simulink model "DCT_2D_BAS2008"  (R2015b)
settings: Solver=VariableStepAuto  StartTime=0.0  StopTime=70*st  RelTol=1e-3
values from neighbouring files (symbols this model uses):
  a = 1    [DCT_2d.m]
  a_mux = 2    [DCT_2d.m]
  st = 10/(10*1e6)    (= 1e-06)    [DCT_2d.m]
libraries: xbsIndex_r4 x169
settings Model: Creator=Namalka  LastModifiedBy=Namalka

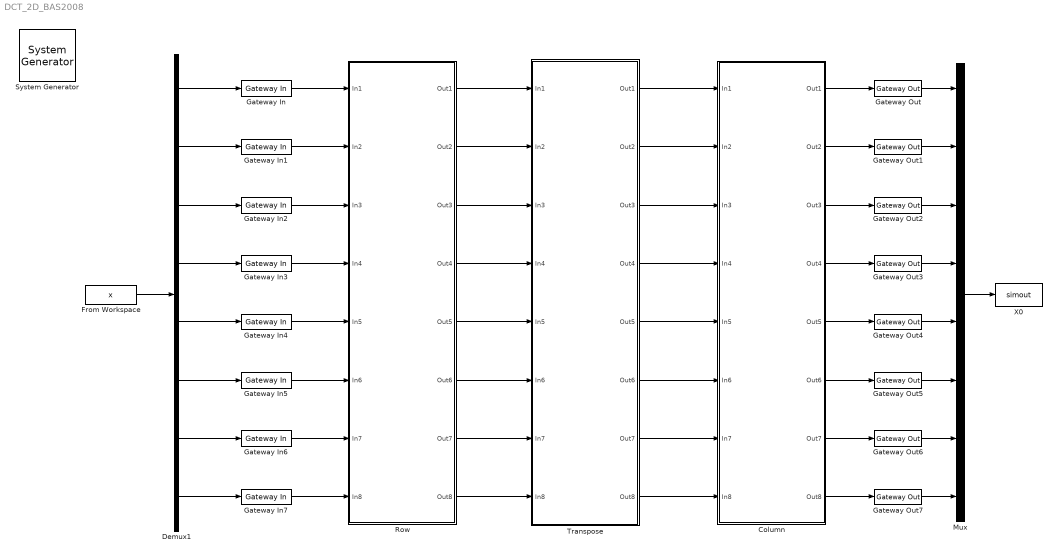
== system DCT_2D_BAS2008 ==
  " System Generator" : xbsIndex_r4/ System Generator  Tag=genX  xilinxfamily=virtex7  part=xc7vx485t  speed=-2  package=ffg1761  synthesis_tool=XST  clock_wrapper=Clock Enables  directory=D:/ISCAS2020/BAS2008/DCT2D  proj_type=Vivado  Synth_file=Vivado Synthesis Defaults  Impl_file=Vivado Implementation Defaults  testbench=off  simulink_period=st  sysclk_period=st*10e6  dcm_input_clock_period=100  incr_netlist=off  trim_vbits=Everywhere in SubSystem  dbl_ovrd=According to Block Masks  core_generation=According to Block Masks  run_coregen=off  deprecated_control=off  eval_field=0  block_type=sysgen
      settings: block_version=10.1
  Column : Subsystem
  Demux1 : Demux  Outputs=8
  From Workspace : FromWorkspace  VariableName=x  SampleTime=0
  Gateway In{,1..7} (8 alike) : xbsIndex_r4/Gateway In  gui_display_data_type=Fixed-point  arith_type="Signed  (2's comp)"  n_bits=W  bin_pt=B  preci_type=Single  exp_width=8  frac_width=24  rows=1  columns=1  quantization="Round  (unbiased: +/- Inf)"  overflow=Saturate  period=st  UseAsADC=off  ADCChannel='1'  interface=None  automatic_assignment=on  address_offset=hex2dec('00')  intf_name=''  intf_description=''  default_value=0  timing_constraint=None  locs_specified=off  LOCs={}  io_standard={}  inherit_from_input=off  hdl_port=on  dbl_ovrd=off  block_type=gatewayin
  Gateway Out{,1..7} (8 alike) : xbsIndex_r4/Gateway Out  inherit_from_input=off  hdl_port=on  rows=1  columns=1  UseAsDAC=off  DACChannel='1'  interface=None  automatic_assignment=on  address_offset=hex2dec('00')  intf_name=''  intf_description=''  timing_constraint=None  locs_specified=off  LOCs={}  io_standard={}  block_type=gatewayout
  Mux : Mux  Inputs=8
  Row : Subsystem
  Transpose : Subsystem
  X0 : ToWorkspace  VariableName=simout  SampleTime=-1
  wires:
  Demux1/1 -> Gateway In/1
  Demux1/2 -> Gateway In1/1
  Demux1/3 -> Gateway In2/1
  Demux1/4 -> Gateway In3/1
  Demux1/5 -> Gateway In4/1
  Demux1/6 -> Gateway In5/1
  Demux1/7 -> Gateway In6/1
  Demux1/8 -> Gateway In7/1
  Gateway In7/1 -> Row/8(In8)
  From Workspace/1 -> Demux1/1
  Gateway In/1 -> Row/1(In1)
  Gateway In6/1 -> Row/7(In7)
  Gateway In1/1 -> Row/2(In2)
  Gateway In2/1 -> Row/3(In3)
  Gateway In3/1 -> Row/4(In4)
  Gateway In4/1 -> Row/5(In5)
  Gateway In5/1 -> Row/6(In6)
  Mux/1 -> X0/1
  Gateway Out7/1 -> Mux/8
  Gateway Out6/1 -> Mux/7
  Gateway Out5/1 -> Mux/6
  Gateway Out4/1 -> Mux/5
  Gateway Out3/1 -> Mux/4
  Gateway Out2/1 -> Mux/3
  Gateway Out1/1 -> Mux/2
  Gateway Out/1 -> Mux/1
  Column/8(Out8) -> Gateway Out7/1
  Column/7(Out7) -> Gateway Out6/1
  Column/1(Out1) -> Gateway Out/1
  Column/2(Out2) -> Gateway Out1/1
  Column/3(Out3) -> Gateway Out2/1
  Column/4(Out4) -> Gateway Out3/1
  Column/6(Out6) -> Gateway Out5/1
  Column/5(Out5) -> Gateway Out4/1
  Transpose/7(Out7) -> Column/7(In7)
  Transpose/1(Out1) -> Column/1(In1)
  Transpose/2(Out2) -> Column/2(In2)
  Transpose/3(Out3) -> Column/3(In3)
  Transpose/4(Out4) -> Column/4(In4)
  Transpose/6(Out6) -> Column/6(In6)
  Transpose/5(Out5) -> Column/5(In5)
  Transpose/8(Out8) -> Column/8(In8)
  Row/7(Out7) -> Transpose/7(In7)
  Row/1(Out1) -> Transpose/1(In1)
  Row/2(Out2) -> Transpose/2(In2)
  Row/3(Out3) -> Transpose/3(In3)
  Row/4(Out4) -> Transpose/4(In4)
  Row/6(Out6) -> Transpose/6(In6)
  Row/5(Out5) -> Transpose/5(In5)
  Row/8(Out8) -> Transpose/8(In8)

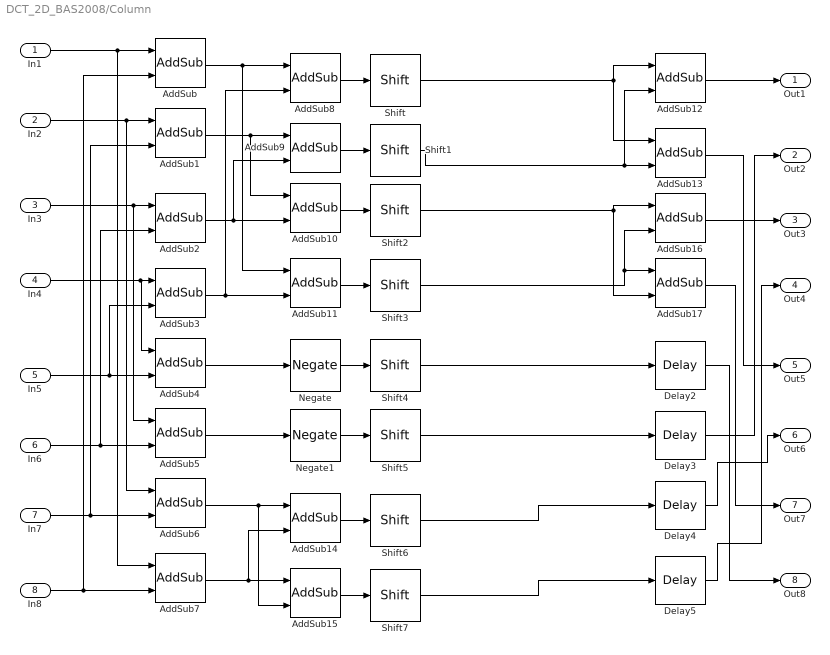
== system DCT_2D_BAS2008/Column ==
  In1 : Inport
  In2 : Inport  Port=2
  In3 : Inport  Port=3
  In4 : Inport  Port=4
  In5 : Inport  Port=5
  In6 : Inport  Port=6
  In7 : Inport  Port=7
  In8 : Inport  Port=8
  AddSub{,1..3,8..9,12,14,16} (9 alike) : xbsIndex_r4/AddSub  mode=Addition  use_carryin=off  use_carryout=off  en=off  latency=a  precision=User Defined  arith_type="Signed  (2's comp)"  n_bits=W  bin_pt=B  quantization="Round  (unbiased: +/- Inf)"  overflow=Saturate  use_behavioral_HDL=off  hw_selection=Fabric  pipelined=off  dbl_ovrd=off  block_type=addsub
  AddSub{4..7,10..11,13,15,17} (9 alike) : xbsIndex_r4/AddSub  mode=Subtraction  use_carryin=off  use_carryout=off  en=off  latency=a  precision=User Defined  arith_type="Signed  (2's comp)"  n_bits=W  bin_pt=B  quantization="Round  (unbiased: +/- Inf)"  overflow=Saturate  use_behavioral_HDL=off  hw_selection=Fabric  pipelined=off  dbl_ovrd=off  block_type=addsub
  Delay{2..5} (4 alike) : xbsIndex_r4/Delay  rst=off  infoeditControl=Selection of Reset will increase slice count due to use of real FFs and instead of SRLs  en=off  latency=a  reg_retiming=off  dbl_ovrd=off  block_type=delay
      settings: infoedit=Hardware notes: A delay line is a chain, each link of which is an SRL16 or SRL32 followed by a flip-flop.
  Negate : xbsIndex_r4/Negate  precision=Full  arith_type=Unsigned  n_bits=16  bin_pt=14  quantization=Truncate  overflow=Wrap  en=off  latency=1  dbl_ovrd=off  block_type=negate
  Negate1 : xbsIndex_r4/Negate  precision=Full  arith_type=Unsigned  n_bits=16  bin_pt=14  quantization=Truncate  overflow=Wrap  en=off  latency=1  dbl_ovrd=off  block_type=negate
  Shift{,1..7} (8 alike) : xbsIndex_r4/Shift  shift_dir=Left  shift_bits=1  en=off  latency=a  precision=Full  arith_type="Signed  (2's comp)"  n_bits=16  bin_pt=14  quantization=Truncate  overflow=Wrap  dbl_ovrd=off  block_type=shift
  Out1 : Outport
  Out2 : Outport  Port=2
  Out3 : Outport  Port=3
  Out4 : Outport  Port=4
  Out5 : Outport  Port=5
  Out6 : Outport  Port=6
  Out7 : Outport  Port=7
  Out8 : Outport  Port=8
  wires:
  In8/1 -> AddSub7/2, AddSub/2
  AddSub8/1 -> Shift/1
  In1/1 -> AddSub/1, AddSub7/1
  In2/1 -> AddSub6/1, AddSub1/1
  In3/1 -> AddSub5/1, AddSub2/1
  In4/1 -> AddSub4/1, AddSub3/1
  In5/1 -> AddSub3/2, AddSub4/2
  In6/1 -> AddSub2/2, AddSub5/2
  In7/1 -> AddSub1/2, AddSub6/2
  AddSub/1 -> AddSub11/1, AddSub8/1
  AddSub1/1 -> AddSub10/1, AddSub9/1
  AddSub2/1 -> AddSub9/2, AddSub10/2
  AddSub3/1 -> AddSub8/2, AddSub11/2
  AddSub9/1 -> Shift1/1
  AddSub11/1 -> Shift3/1
  AddSub4/1 -> Negate/1
  AddSub5/1 -> Negate1/1
  AddSub10/1 -> Shift2/1
  Negate/1 -> Shift4/1
  Negate1/1 -> Shift5/1
  AddSub6/1 -> AddSub15/2, AddSub14/1
  AddSub7/1 -> AddSub15/1, AddSub14/2
  Shift/1 -> AddSub13/1, AddSub12/1
  Shift1/1 -> AddSub12/2, AddSub13/2
  Shift4/1 -> Delay2/1
  Shift5/1 -> Delay3/1
  AddSub14/1 -> Shift6/1
  AddSub15/1 -> Shift7/1
  Shift2/1 -> AddSub17/2, AddSub16/1
  Shift3/1 -> AddSub17/1, AddSub16/2
  AddSub12/1 -> Out1/1
  Shift6/1 -> Delay4/1
  Shift7/1 -> Delay5/1
  AddSub13/1 -> Out5/1
  AddSub16/1 -> Out3/1
  AddSub17/1 -> Out7/1
  Delay2/1 -> Out8/1
  Delay3/1 -> Out2/1
  Delay4/1 -> Out6/1
  Delay5/1 -> Out4/1

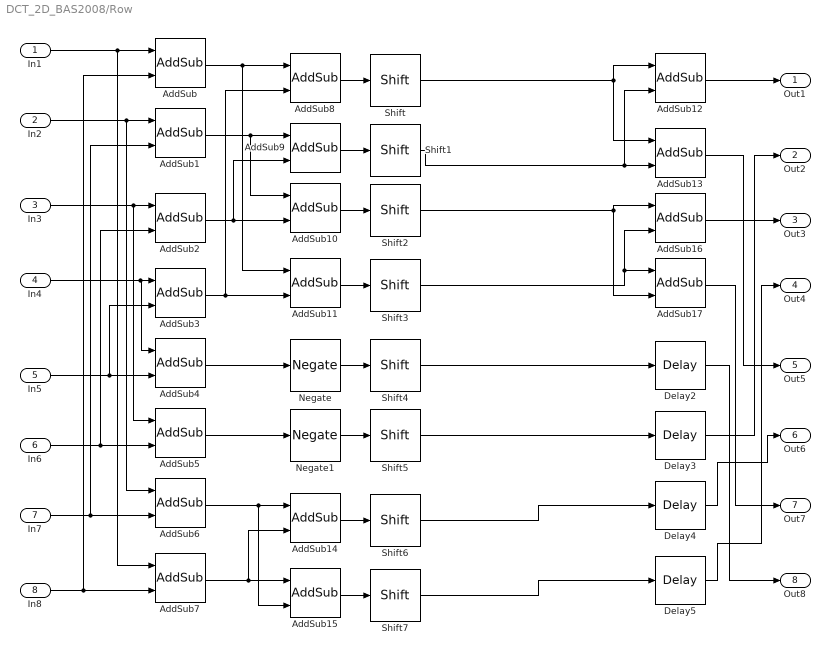
== system DCT_2D_BAS2008/Row ==
  In1 : Inport
  In2 : Inport  Port=2
  In3 : Inport  Port=3
  In4 : Inport  Port=4
  In5 : Inport  Port=5
  In6 : Inport  Port=6
  In7 : Inport  Port=7
  In8 : Inport  Port=8
  AddSub{,1..3,8..9,12,14,16} (9 alike) : xbsIndex_r4/AddSub  mode=Addition  use_carryin=off  use_carryout=off  en=off  latency=a  precision=User Defined  arith_type="Signed  (2's comp)"  n_bits=W  bin_pt=B  quantization="Round  (unbiased: +/- Inf)"  overflow=Saturate  use_behavioral_HDL=off  hw_selection=Fabric  pipelined=off  dbl_ovrd=off  block_type=addsub
  AddSub{4..7,10..11,13,15,17} (9 alike) : xbsIndex_r4/AddSub  mode=Subtraction  use_carryin=off  use_carryout=off  en=off  latency=a  precision=User Defined  arith_type="Signed  (2's comp)"  n_bits=W  bin_pt=B  quantization="Round  (unbiased: +/- Inf)"  overflow=Saturate  use_behavioral_HDL=off  hw_selection=Fabric  pipelined=off  dbl_ovrd=off  block_type=addsub
  Delay{2..5} (4 alike) : xbsIndex_r4/Delay  rst=off  infoeditControl=Selection of Reset will increase slice count due to use of real FFs and instead of SRLs  en=off  latency=a  reg_retiming=off  dbl_ovrd=off  block_type=delay
      settings: infoedit=Hardware notes: A delay line is a chain, each link of which is an SRL16 or SRL32 followed by a flip-flop.
  Negate : xbsIndex_r4/Negate  precision=Full  arith_type=Unsigned  n_bits=16  bin_pt=14  quantization=Truncate  overflow=Wrap  en=off  latency=1  dbl_ovrd=off  block_type=negate
  Negate1 : xbsIndex_r4/Negate  precision=Full  arith_type=Unsigned  n_bits=16  bin_pt=14  quantization=Truncate  overflow=Wrap  en=off  latency=1  dbl_ovrd=off  block_type=negate
  Shift{,1..7} (8 alike) : xbsIndex_r4/Shift  shift_dir=Left  shift_bits=1  en=off  latency=a  precision=Full  arith_type="Signed  (2's comp)"  n_bits=16  bin_pt=14  quantization=Truncate  overflow=Wrap  dbl_ovrd=off  block_type=shift
  Out1 : Outport
  Out2 : Outport  Port=2
  Out3 : Outport  Port=3
  Out4 : Outport  Port=4
  Out5 : Outport  Port=5
  Out6 : Outport  Port=6
  Out7 : Outport  Port=7
  Out8 : Outport  Port=8
  wires:
  In8/1 -> AddSub7/2, AddSub/2
  AddSub8/1 -> Shift/1
  In1/1 -> AddSub/1, AddSub7/1
  In2/1 -> AddSub6/1, AddSub1/1
  In3/1 -> AddSub5/1, AddSub2/1
  In4/1 -> AddSub4/1, AddSub3/1
  In5/1 -> AddSub3/2, AddSub4/2
  In6/1 -> AddSub2/2, AddSub5/2
  In7/1 -> AddSub1/2, AddSub6/2
  AddSub/1 -> AddSub11/1, AddSub8/1
  AddSub1/1 -> AddSub10/1, AddSub9/1
  AddSub2/1 -> AddSub9/2, AddSub10/2
  AddSub3/1 -> AddSub8/2, AddSub11/2
  AddSub9/1 -> Shift1/1
  AddSub11/1 -> Shift3/1
  AddSub4/1 -> Negate/1
  AddSub5/1 -> Negate1/1
  AddSub10/1 -> Shift2/1
  Negate/1 -> Shift4/1
  Negate1/1 -> Shift5/1
  AddSub6/1 -> AddSub15/2, AddSub14/1
  AddSub7/1 -> AddSub15/1, AddSub14/2
  Shift/1 -> AddSub13/1, AddSub12/1
  Shift1/1 -> AddSub12/2, AddSub13/2
  Shift4/1 -> Delay2/1
  Shift5/1 -> Delay3/1
  AddSub14/1 -> Shift6/1
  AddSub15/1 -> Shift7/1
  Shift2/1 -> AddSub17/2, AddSub16/1
  Shift3/1 -> AddSub17/1, AddSub16/2
  AddSub12/1 -> Out1/1
  Shift6/1 -> Delay4/1
  Shift7/1 -> Delay5/1
  AddSub13/1 -> Out5/1
  AddSub16/1 -> Out3/1
  AddSub17/1 -> Out7/1
  Delay2/1 -> Out8/1
  Delay3/1 -> Out2/1
  Delay4/1 -> Out6/1
  Delay5/1 -> Out4/1

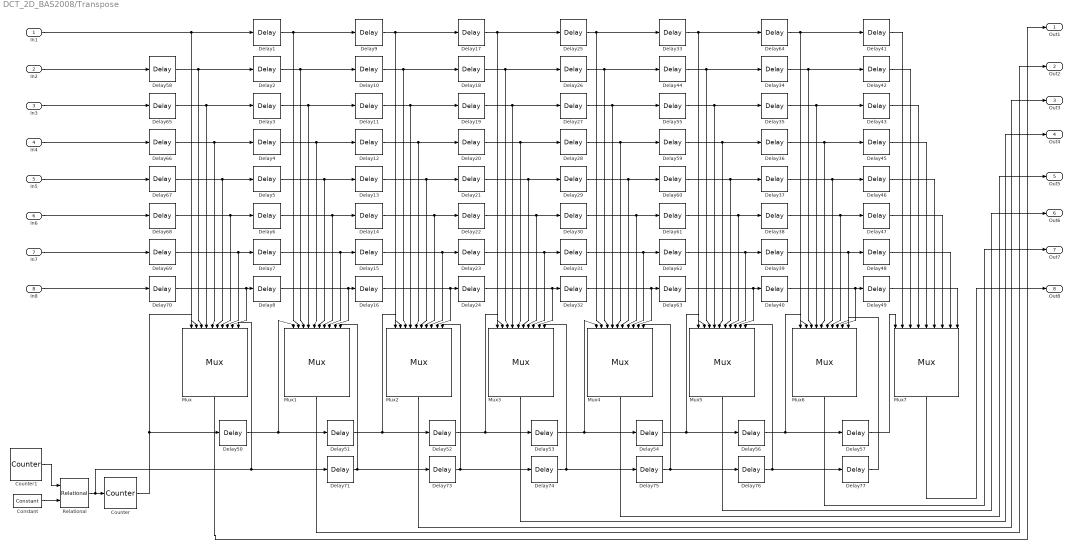
== system DCT_2D_BAS2008/Transpose ==
  In1 : Inport
  In2 : Inport  Port=2
  In3 : Inport  Port=3
  In4 : Inport  Port=4
  In5 : Inport  Port=5
  In6 : Inport  Port=6
  In7 : Inport  Port=7
  In8 : Inport  Port=8
  Constant : xbsIndex_r4/Constant  const=2  gui_display_data_type=Fixed-point  arith_type=Signed (2's comp)  n_bits=8  bin_pt=0  preci_type=Single  exp_width=8  frac_width=24  explicit_period=on  period=st  equ=P=C  opselect=C  inp2=PCIN>>17  opr=+  inp1=P  carry=CIN  dbl_ovrd=off  block_type=constant
  Counter : xbsIndex_r4/Counter  cnt_type=Count Limited  cnt_to=7  operation=Up  start_count=0  cnt_by_val=1  arith_type=Unsigned  n_bits=3  bin_pt=0  load_pin=off  rst=off  en=on  explicit_period=on  period=st  use_behavioral_HDL=off  implementation=Fabric  dbl_ovrd=off  block_type=counter
  Counter1 : xbsIndex_r4/Counter  cnt_type=Free Running  cnt_to=Inf  operation=Up  start_count=0  cnt_by_val=1  arith_type=Unsigned  n_bits=8  bin_pt=0  load_pin=off  rst=off  en=off  explicit_period=on  period=st  use_behavioral_HDL=off  implementation=Fabric  dbl_ovrd=off  block_type=counter
  Delay{1..49,55,58..64,73..77} (62 alike) : xbsIndex_r4/Delay  rst=off  infoeditControl=Selection of Reset will increase slice count due to use of real FFs and instead of SRLs  en=off  latency=a  reg_retiming=off  dbl_ovrd=off  block_type=delay
      settings: infoedit=Hardware notes: A delay line is a chain, each link of which is an SRL16 or SRL32 followed by a flip-flop.
  Delay{50..54,56..57} (7 alike) : xbsIndex_r4/Delay  rst=off  infoeditControl=Selection of Reset will increase slice count due to use of real FFs and instead of SRLs  en=off  latency=b  reg_retiming=off  dbl_ovrd=off  block_type=delay
      settings: infoedit=Hardware notes: A delay line is a chain, each link of which is an SRL16 or SRL32 followed by a flip-flop.
  Delay65 : xbsIndex_r4/Delay  rst=off  infoeditControl=Selection of Reset will increase slice count due to use of real FFs and instead of SRLs  en=off  latency=2*a  reg_retiming=off  dbl_ovrd=off  block_type=delay
      settings: infoedit=Hardware notes: A delay line is a chain, each link of which is an SRL16 or SRL32 followed by a flip-flop.
  Delay66 : xbsIndex_r4/Delay  rst=off  infoeditControl=Selection of Reset will increase slice count due to use of real FFs and instead of SRLs  en=off  latency=3*a  reg_retiming=off  dbl_ovrd=off  block_type=delay
      settings: infoedit=Hardware notes: A delay line is a chain, each link of which is an SRL16 or SRL32 followed by a flip-flop.
  Delay67 : xbsIndex_r4/Delay  rst=off  infoeditControl=Selection of Reset will increase slice count due to use of real FFs and instead of SRLs  en=off  latency=4*a  reg_retiming=off  dbl_ovrd=off  block_type=delay
      settings: infoedit=Hardware notes: A delay line is a chain, each link of which is an SRL16 or SRL32 followed by a flip-flop.
  Delay68 : xbsIndex_r4/Delay  rst=off  infoeditControl=Selection of Reset will increase slice count due to use of real FFs and instead of SRLs  en=off  latency=5*a  reg_retiming=off  dbl_ovrd=off  block_type=delay
      settings: infoedit=Hardware notes: A delay line is a chain, each link of which is an SRL16 or SRL32 followed by a flip-flop.
  Delay69 : xbsIndex_r4/Delay  rst=off  infoeditControl=Selection of Reset will increase slice count due to use of real FFs and instead of SRLs  en=off  latency=6*a  reg_retiming=off  dbl_ovrd=off  block_type=delay
      settings: infoedit=Hardware notes: A delay line is a chain, each link of which is an SRL16 or SRL32 followed by a flip-flop.
  Delay70 : xbsIndex_r4/Delay  rst=off  infoeditControl=Selection of Reset will increase slice count due to use of real FFs and instead of SRLs  en=off  latency=7*a  reg_retiming=off  dbl_ovrd=off  block_type=delay
      settings: infoedit=Hardware notes: A delay line is a chain, each link of which is an SRL16 or SRL32 followed by a flip-flop.
  Delay71 : xbsIndex_r4/Delay  rst=off  infoeditControl=Selection of Reset will increase slice count due to use of real FFs and instead of SRLs  en=off  latency=2*a  reg_retiming=off  dbl_ovrd=off  block_type=delay
      settings: infoedit=Hardware notes: A delay line is a chain, each link of which is an SRL16 or SRL32 followed by a flip-flop.
  Mux : xbsIndex_r4/Mux  inputs=8  en=on  latency=7*a_mux  precision=User Defined  arith_type="Signed  (2's comp)"  n_bits=8  bin_pt=0  quantization="Round  (unbiased: +/- Inf)"  overflow=Saturate  dbl_ovrd=off  block_type=mux
  Mux1 : xbsIndex_r4/Mux  inputs=8  en=on  latency=6*a_mux  precision=User Defined  arith_type="Signed  (2's comp)"  n_bits=8  bin_pt=0  quantization="Round  (unbiased: +/- Inf)"  overflow=Saturate  dbl_ovrd=off  block_type=mux
  Mux2 : xbsIndex_r4/Mux  inputs=8  en=on  latency=5*a_mux  precision=User Defined  arith_type="Signed  (2's comp)"  n_bits=8  bin_pt=0  quantization="Round  (unbiased: +/- Inf)"  overflow=Saturate  dbl_ovrd=off  block_type=mux
  Mux3 : xbsIndex_r4/Mux  inputs=8  en=on  latency=4*a_mux  precision=User Defined  arith_type="Signed  (2's comp)"  n_bits=8  bin_pt=0  quantization="Round  (unbiased: +/- Inf)"  overflow=Saturate  dbl_ovrd=off  block_type=mux
  Mux4 : xbsIndex_r4/Mux  inputs=8  en=on  latency=3*a_mux  precision=User Defined  arith_type="Signed  (2's comp)"  n_bits=8  bin_pt=0  quantization="Round  (unbiased: +/- Inf)"  overflow=Saturate  dbl_ovrd=off  block_type=mux
  Mux5 : xbsIndex_r4/Mux  inputs=8  en=on  latency=2*a_mux  precision=User Defined  arith_type="Signed  (2's comp)"  n_bits=8  bin_pt=0  quantization="Round  (unbiased: +/- Inf)"  overflow=Saturate  dbl_ovrd=off  block_type=mux
  Mux6 : xbsIndex_r4/Mux  inputs=8  en=on  latency=a_mux  precision=User Defined  arith_type="Signed  (2's comp)"  n_bits=8  bin_pt=0  quantization="Round  (unbiased: +/- Inf)"  overflow=Saturate  dbl_ovrd=off  block_type=mux
  Mux7 : xbsIndex_r4/Mux  inputs=8  en=off  latency=1  precision=User Defined  arith_type="Signed  (2's comp)"  n_bits=8  bin_pt=0  quantization="Round  (unbiased: +/- Inf)"  overflow=Saturate  dbl_ovrd=off  block_type=mux
  Relational : xbsIndex_r4/Relational  mode=a>b  op_type=Bool  en=off  latency=a  dbl_ovrd=off  block_type=relational
  Out1 : Outport
  Out2 : Outport  Port=2
  Out3 : Outport  Port=3
  Out4 : Outport  Port=4
  Out5 : Outport  Port=5
  Out6 : Outport  Port=6
  Out7 : Outport  Port=7
  Out8 : Outport  Port=8
  wires:
  In8/1 -> Delay70/1
  In5/1 -> Delay67/1
  In6/1 -> Delay68/1
  In7/1 -> Delay69/1
  In1/1 -> Mux/2, Delay1/1
  In2/1 -> Delay58/1
  In4/1 -> Delay66/1
  In3/1 -> Delay65/1
  Delay8/1 -> Mux1/9, Delay16/1
  Delay5/1 -> Mux1/6, Delay13/1
  Delay6/1 -> Mux1/7, Delay14/1
  Delay7/1 -> Mux1/8, Delay15/1
  Delay1/1 -> Mux1/2, Delay9/1
  Delay2/1 -> Mux1/3, Delay10/1
  Delay4/1 -> Delay12/1, Mux1/5
  Delay3/1 -> Mux1/4, Delay11/1
  Delay16/1 -> Mux2/9, Delay24/1
  Delay13/1 -> Mux2/6, Delay21/1
  Delay14/1 -> Mux2/7, Delay22/1
  Delay15/1 -> Mux2/8, Delay23/1
  Delay9/1 -> Mux2/2, Delay17/1
  Delay10/1 -> Mux2/3, Delay18/1
  Delay12/1 -> Delay20/1, Mux2/5
  Delay11/1 -> Mux2/4, Delay19/1
  Delay24/1 -> Mux3/9, Delay32/1
  Delay21/1 -> Mux3/6, Delay29/1
  Delay22/1 -> Mux3/7, Delay30/1
  Delay23/1 -> Mux3/8, Delay31/1
  Delay17/1 -> Mux3/2, Delay25/1
  Delay18/1 -> Mux3/3, Delay26/1
  Delay20/1 -> Delay28/1, Mux3/5
  Delay19/1 -> Mux3/4, Delay27/1
  Delay32/1 -> Mux4/9, Delay63/1
  Delay29/1 -> Mux4/6, Delay60/1
  Delay30/1 -> Mux4/7, Delay61/1
  Delay31/1 -> Mux4/8, Delay62/1
  Delay25/1 -> Mux4/2, Delay33/1
  Delay26/1 -> Mux4/3, Delay44/1
  Delay28/1 -> Delay59/1, Mux4/5
  Delay27/1 -> Mux4/4, Delay55/1
  Delay63/1 -> Mux5/9, Delay40/1
  Delay60/1 -> Mux5/6, Delay37/1
  Delay61/1 -> Mux5/7, Delay38/1
  Delay62/1 -> Mux5/8, Delay39/1
  Delay33/1 -> Mux5/2, Delay64/1
  Delay44/1 -> Mux5/3, Delay34/1
  Delay59/1 -> Delay36/1, Mux5/5
  Delay55/1 -> Mux5/4, Delay35/1
  Delay40/1 -> Mux6/9, Delay49/1
  Delay37/1 -> Mux6/6, Delay46/1
  Delay38/1 -> Mux6/7, Delay47/1
  Delay39/1 -> Mux6/8, Delay48/1
  Delay64/1 -> Mux6/2, Delay41/1
  Delay34/1 -> Mux6/3, Delay42/1
  Delay36/1 -> Delay45/1, Mux6/5
  Delay35/1 -> Mux6/4, Delay43/1
  Delay49/1 -> Mux7/9
  Delay46/1 -> Mux7/6
  Delay47/1 -> Mux7/7
  Delay48/1 -> Mux7/8
  Delay41/1 -> Mux7/2
  Delay42/1 -> Mux7/3
  Delay45/1 -> Mux7/5
  Delay43/1 -> Mux7/4
  Mux6/1 -> Out7/1
  Mux5/1 -> Out6/1
  Mux4/1 -> Out5/1
  Mux3/1 -> Out4/1
  Mux2/1 -> Out3/1
  Mux1/1 -> Out2/1
  Delay50/1 -> Delay51/1, Mux1/1
  Delay51/1 -> Delay52/1, Mux2/1
  Delay52/1 -> Delay53/1, Mux3/1
  Delay53/1 -> Delay54/1, Mux4/1
  Delay54/1 -> Delay56/1, Mux5/1
  Delay56/1 -> Delay57/1, Mux6/1
  Delay58/1 -> Mux/3, Delay2/1
  Delay65/1 -> Mux/4, Delay3/1
  Delay66/1 -> Delay4/1, Mux/5
  Delay67/1 -> Mux/6, Delay5/1
  Delay68/1 -> Mux/7, Delay6/1
  Delay69/1 -> Mux/8, Delay7/1
  Delay70/1 -> Mux/9, Delay8/1
  Counter1/1 -> Relational/1
  Constant/1 -> Relational/2
  Counter/1 -> Mux/1, Delay50/1
  Mux/1 -> Out1/1
  Mux7/1 -> Out8/1
  Delay57/1 -> Mux7/1
  Delay71/1 -> Mux1/10, Delay73/1
  Relational/1 -> Delay71/1, Mux/10, Counter/1
  Delay73/1 -> Delay74/1, Mux2/10
  Delay74/1 -> Delay75/1, Mux3/10
  Delay75/1 -> Mux4/10, Delay76/1
  Delay76/1 -> Mux5/10, Delay77/1
  Delay77/1 -> Mux6/10
